simulink model "adc5g_r2_counter"  (Simulink 7.6)
settings: Solver=ode45  StartTime=0.0  StopTime=10.0  RelTol=1e-3
libraries: xbsIndex_r4 x22, simulink x16, dspsigops x16, xps_library x2, casper_library_misc x1
settings Model: Creator=rprimian  LastModifiedBy=rprimian
settings DebuggingCC: SolverPrmCheckMsg=none  StrictBusMsg=Warning

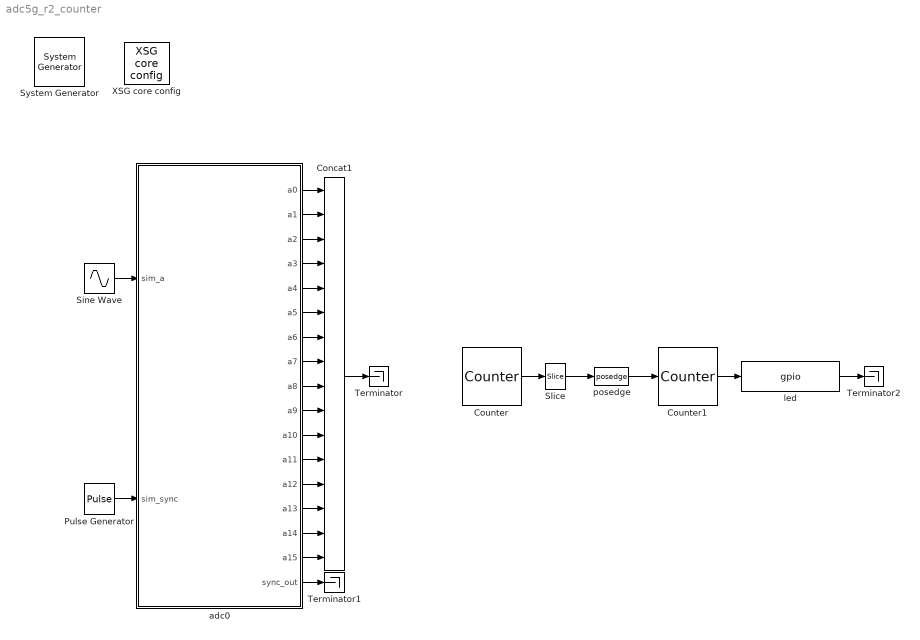
== system adc5g_r2_counter ==
  " System Generator" : xbsIndex_r4/ System Generator  Tag=genX  SystemSampleTime=-1  xilinxfamily=virtex6  part=xc6vsx475t  speed=-1  package=ff1759  synthesis_tool=XST  clock_wrapper=Clock Enables  directory=./adc5g_r2_counter/sysgen  proj_type=Project Navigator  testbench=off  simulink_period=1  sysclk_period=8  dcm_input_clock_period=100  incr_netlist=off  trim_vbits=Everywhere in SubSystem  dbl_ovrd=According to Block Masks  core_generation=According to Block Masks  run_coregen=off  deprecated_control=off  eval_field=0  block_type=sysgen
      settings: block_version=11.4
  Concat1 : xbsIndex_r4/Concat  num_inputs=16  dbl_ovrd=off  block_type=concat
  Counter : xbsIndex_r4/Counter  cnt_type=Free Running  cnt_to=Inf  operation=Up  start_count=0  cnt_by_val=1  arith_type=Unsigned  n_bits=32  bin_pt=0  load_pin=off  rst=off  en=off  explicit_period=on  period=1  dbl_ovrd=off  use_behavioral_HDL=off  implementation=Fabric  block_type=counter
  Counter1 : xbsIndex_r4/Counter  cnt_type=Free Running  cnt_to=Inf  operation=Up  start_count=0  cnt_by_val=1  arith_type=Unsigned  n_bits=8  bin_pt=0  load_pin=off  rst=off  en=on  explicit_period=on  period=1  dbl_ovrd=off  use_behavioral_HDL=off  implementation=Fabric  block_type=counter
  Pulse Generator : DiscretePulseGenerator  Period=1000
  Sine Wave : Sin  SineType=Sample based  SampleTime=1/8
  Slice : xbsIndex_r4/Slice  nbits=1  boolean_output=on  mode=Upper Bit Location + Width  bit1=-2  base1=MSB of Input  bit0=0  base0=LSB of Input  dbl_ovrd=off  block_type=slice
  Terminator : Terminator
  Terminator1 : Terminator
  Terminator2 : Terminator
  XSG core config : xps_library/XSG core config  Tag=xps:xsg  SystemSampleTime=-1  hw_sys=ROACH2:sx475t  ibob_linux=off  clk_src=adc0_clk  iBOB_clk_src=sys_clk  BEE2_ctrl_clk_src=sys_clk  BEE2_usr_clk_src=sys_clk  ROACH_clk_src=adc0_clk  ROACH2_clk_src=adc0_clk  CORR_clk_src=sys_clk  gpio_clk_io_group=iBOB:sma  gpio_clk_bit_index=0  clk_rate=125  sample_period=1  synthesis_tool=XST  mpc_type=powerpc440_ext
  adc0 : Subsystem  Tag=xps:adc5g  AncestorBlock=xps_library/ADCs/asiaa_adc5g  mask(adc5g){input_mode=One-channel -- A, adc_brd=ZDOK 0, demux=1:1, adc_bit_width=8, adc_clk_rate=1000, using_ctrl=on, test_ramp=off}
      mask prompts: input_mode "Input mode:"; adc_brd "ADC Board"; demux "Internal demux"; adc_bit_width "ADC Resolution (bits):"; adc_clk_rate "ADC Clock Rate (MHz):"; using_ctrl "use control"; test_ramp "start in test ramp mode"
      mask help:
      | Interface for the ASIAA 5 GSps ADC. Supports interleaving all four
      | cores using either input A or C, or interleaving two-cores each for
      | A and C. The hardware itself comes in two versions:
      |
      | DMUX 1:2 -- 4-bit samples, 4 parallel streams
      | DMUX 1:1 -- 8-bit samples, 2 parallel streams
      |
      | In either configuration this block will output 8 parallel streams
      | but the underlying interface, and the bitwidth of the samples,
      | will be different.
      mask init:
      | adc5g_init(gcb,...
      |     'input_mode', input_mode,...
      |     'demux', demux,...
      |     'adc_clk_rate', adc_clk_rate,...
      |     'adc_bit_width', adc_bit_width,...
      |     'adc_brd', adc_brd,...
      |     'using_ctrl', using_ctrl,...
      |     'test_ramp', test_ramp);
      mask StyleString: popup(One-channel -- A|One-channel -- C|Two-channel -- A&C),popup(ZDOK 0|ZDOK 1),popup(1:1|1:2),edit,edit,checkbox,checkbox
      mask CallbackString:
      | ||demux = get_param(gcb,'demux');
      | if(strcmp(demux,'1:1')),
      |     set_param(gcb, 'adc_bit_width', '8')
      | elseif(strcmp(demux, '1:2')),
      |     set_param(gcb, 'adc_bit_width', '4');
      | else
      | end||||
  led : xps_library/gpio  Tag=xps:gpio  SystemSampleTime=-1  io_group=ROACH2:led  io_dir=out  arith_type=Unsigned  bitwidth=8  bin_pt=0  bit_index=[0 1 2 3 4 5 6 7]  sample_period=1  use_single_ended=off  use_ddr=off  reg_iob=on  reg_clk_phase=0  termination=None
      link override convert: arith_type=Boolean  n_bits=8  bin_pt=0
  posedge : casper_library_misc/posedge  Tag=Rising Edge Detector  SystemSampleTime=-1
  wires:
  Pulse Generator/1 -> adc0/2(sim_sync)
  Concat1/1 -> Terminator/1
  Sine Wave/1 -> adc0/1(sim_a)
  adc0/1(a0) -> Concat1/1
  adc0/2(a1) -> Concat1/2
  adc0/3(a2) -> Concat1/3
  adc0/4(a3) -> Concat1/4
  adc0/5(a4) -> Concat1/5
  adc0/6(a5) -> Concat1/6
  adc0/7(a6) -> Concat1/7
  adc0/8(a7) -> Concat1/8
  adc0/9(a8) -> Concat1/9
  adc0/10(a9) -> Concat1/10
  adc0/11(a10) -> Concat1/11
  adc0/12(a11) -> Concat1/12
  adc0/13(a12) -> Concat1/13
  adc0/14(a13) -> Concat1/14
  adc0/15(a14) -> Concat1/15
  adc0/16(a15) -> Concat1/16
  adc0/17(sync_out) -> Terminator1/1
  Counter/1 -> Slice/1
  Slice/1 -> posedge/1
  led/1 -> Terminator2/1
  Counter1/1 -> led/1
  posedge/1 -> Counter1/1

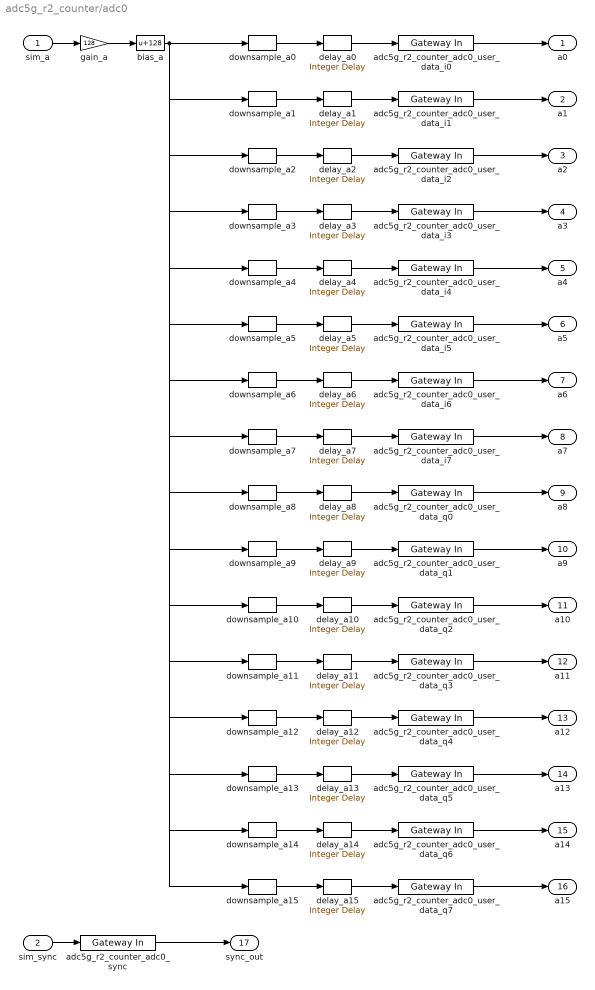
== system adc5g_r2_counter/adc0 ==
  sim_a : Inport
  sim_sync : Inport  Port=2
  adc5g_r2_counter_adc0_sync : xbsIndex_r4/Gateway In  arith_type=Boolean  n_bits=16  bin_pt=14  quantization="Round  (unbiased: +/- Inf)"  overflow=Saturate  period=1  dbl_ovrd=off  timing_constraint=None  locs_specified=off  LOCs={}  hdl_port=on  block_type=gatewayin
      settings: infoedit="Gateway in block.  Converts inputs of type Simulink integer, double and fixed point to  Xilinx fixed point type.<br><br>Hardware notes:  In hardware these blocks become top level input ports."
  adc5g_r2_counter_adc0_user_data_i{0..7} (8 alike) : xbsIndex_r4/Gateway In  arith_type=Unsigned  n_bits=8  bin_pt=0  quantization=Truncate  overflow=Wrap  period=1  dbl_ovrd=off  timing_constraint=None  locs_specified=off  LOCs={}  hdl_port=on  block_type=gatewayin
      settings: infoedit="Gateway in block.  Converts inputs of type Simulink integer, double and fixed point to  Xilinx fixed point type.<br><br>Hardware notes:  In hardware these blocks become top level input ports."
  adc5g_r2_counter_adc0_user_data_q{0..7} (8 alike) : xbsIndex_r4/Gateway In  arith_type=Unsigned  n_bits=8  bin_pt=0  quantization=Truncate  overflow=Wrap  period=1  dbl_ovrd=off  timing_constraint=None  locs_specified=off  LOCs={}  hdl_port=on  block_type=gatewayin
      settings: infoedit="Gateway in block.  Converts inputs of type Simulink integer, double and fixed point to  Xilinx fixed point type.<br><br>Hardware notes:  In hardware these blocks become top level input ports."
  bias_a : Bias  Bias=128  SaturateOnIntegerOverflow=on
  delay_a0 : simulink/Discrete/Integer Delay  NumDelays=2  InputProcessing=Inherited  vinit=0  samptime=-1
  delay_a{1..15} (15 alike) : simulink/Discrete/Integer Delay  NumDelays=1  InputProcessing=Inherited  vinit=0  samptime=-1
  downsample_a0 : dspsigops/Downsample  N=16  phase=0  InputProcessing=Inherited (this choice will be removed - see release notes)  RateOptions=Enforce single-rate processing  smode=Allow multirate  fmode=Maintain input frame size  ic=0
  downsample_a1 : dspsigops/Downsample  N=16  phase=1  InputProcessing=Inherited (this choice will be removed - see release notes)  RateOptions=Enforce single-rate processing  smode=Allow multirate  fmode=Maintain input frame size  ic=0
  downsample_a10 : dspsigops/Downsample  N=16  phase=10  InputProcessing=Inherited (this choice will be removed - see release notes)  RateOptions=Enforce single-rate processing  smode=Allow multirate  fmode=Maintain input frame size  ic=0
  downsample_a11 : dspsigops/Downsample  N=16  phase=11  InputProcessing=Inherited (this choice will be removed - see release notes)  RateOptions=Enforce single-rate processing  smode=Allow multirate  fmode=Maintain input frame size  ic=0
  downsample_a12 : dspsigops/Downsample  N=16  phase=12  InputProcessing=Inherited (this choice will be removed - see release notes)  RateOptions=Enforce single-rate processing  smode=Allow multirate  fmode=Maintain input frame size  ic=0
  downsample_a13 : dspsigops/Downsample  N=16  phase=13  InputProcessing=Inherited (this choice will be removed - see release notes)  RateOptions=Enforce single-rate processing  smode=Allow multirate  fmode=Maintain input frame size  ic=0
  downsample_a14 : dspsigops/Downsample  N=16  phase=14  InputProcessing=Inherited (this choice will be removed - see release notes)  RateOptions=Enforce single-rate processing  smode=Allow multirate  fmode=Maintain input frame size  ic=0
  downsample_a15 : dspsigops/Downsample  N=16  phase=15  InputProcessing=Inherited (this choice will be removed - see release notes)  RateOptions=Enforce single-rate processing  smode=Allow multirate  fmode=Maintain input frame size  ic=0
  downsample_a2 : dspsigops/Downsample  N=16  phase=2  InputProcessing=Inherited (this choice will be removed - see release notes)  RateOptions=Enforce single-rate processing  smode=Allow multirate  fmode=Maintain input frame size  ic=0
  downsample_a3 : dspsigops/Downsample  N=16  phase=3  InputProcessing=Inherited (this choice will be removed - see release notes)  RateOptions=Enforce single-rate processing  smode=Allow multirate  fmode=Maintain input frame size  ic=0
  downsample_a4 : dspsigops/Downsample  N=16  phase=4  InputProcessing=Inherited (this choice will be removed - see release notes)  RateOptions=Enforce single-rate processing  smode=Allow multirate  fmode=Maintain input frame size  ic=0
  downsample_a5 : dspsigops/Downsample  N=16  phase=5  InputProcessing=Inherited (this choice will be removed - see release notes)  RateOptions=Enforce single-rate processing  smode=Allow multirate  fmode=Maintain input frame size  ic=0
  downsample_a6 : dspsigops/Downsample  N=16  phase=6  InputProcessing=Inherited (this choice will be removed - see release notes)  RateOptions=Enforce single-rate processing  smode=Allow multirate  fmode=Maintain input frame size  ic=0
  downsample_a7 : dspsigops/Downsample  N=16  phase=7  InputProcessing=Inherited (this choice will be removed - see release notes)  RateOptions=Enforce single-rate processing  smode=Allow multirate  fmode=Maintain input frame size  ic=0
  downsample_a8 : dspsigops/Downsample  N=16  phase=8  InputProcessing=Inherited (this choice will be removed - see release notes)  RateOptions=Enforce single-rate processing  smode=Allow multirate  fmode=Maintain input frame size  ic=0
  downsample_a9 : dspsigops/Downsample  N=16  phase=9  InputProcessing=Inherited (this choice will be removed - see release notes)  RateOptions=Enforce single-rate processing  smode=Allow multirate  fmode=Maintain input frame size  ic=0
  gain_a : Gain  Gain=128  SaturateOnIntegerOverflow=on  OutDataTypeStr=Inherit: Same as input  ParamDataTypeStr=Inherit: Same as input
  a0 : Outport
  a1 : Outport  Port=2
  a2 : Outport  Port=3
  a3 : Outport  Port=4
  a4 : Outport  Port=5
  a5 : Outport  Port=6
  a6 : Outport  Port=7
  a7 : Outport  Port=8
  a8 : Outport  Port=9
  a9 : Outport  Port=10
  a10 : Outport  Port=11
  a11 : Outport  Port=12
  a12 : Outport  Port=13
  a13 : Outport  Port=14
  a14 : Outport  Port=15
  a15 : Outport  Port=16
  sync_out : Outport  Port=17
  wires:
  sim_a/1 -> gain_a/1
  gain_a/1 -> bias_a/1
  bias_a/1 -> downsample_a0/1, downsample_a1/1, downsample_a2/1, downsample_a3/1, downsample_a4/1, downsample_a5/1, downsample_a6/1, downsample_a7/1, downsample_a8/1, downsample_a9/1, downsample_a10/1, downsample_a11/1, downsample_a12/1, downsample_a13/1, downsample_a14/1, downsample_a15/1
  downsample_a0/1 -> delay_a0/1
  delay_a0/1 -> adc5g_r2_counter_adc0_user_data_i0/1
  adc5g_r2_counter_adc0_user_data_i0/1 -> a0/1
  downsample_a1/1 -> delay_a1/1
  delay_a1/1 -> adc5g_r2_counter_adc0_user_data_i1/1
  adc5g_r2_counter_adc0_user_data_i1/1 -> a1/1
  downsample_a2/1 -> delay_a2/1
  delay_a2/1 -> adc5g_r2_counter_adc0_user_data_i2/1
  adc5g_r2_counter_adc0_user_data_i2/1 -> a2/1
  downsample_a3/1 -> delay_a3/1
  delay_a3/1 -> adc5g_r2_counter_adc0_user_data_i3/1
  adc5g_r2_counter_adc0_user_data_i3/1 -> a3/1
  downsample_a4/1 -> delay_a4/1
  delay_a4/1 -> adc5g_r2_counter_adc0_user_data_i4/1
  adc5g_r2_counter_adc0_user_data_i4/1 -> a4/1
  downsample_a5/1 -> delay_a5/1
  delay_a5/1 -> adc5g_r2_counter_adc0_user_data_i5/1
  adc5g_r2_counter_adc0_user_data_i5/1 -> a5/1
  downsample_a6/1 -> delay_a6/1
  delay_a6/1 -> adc5g_r2_counter_adc0_user_data_i6/1
  adc5g_r2_counter_adc0_user_data_i6/1 -> a6/1
  downsample_a7/1 -> delay_a7/1
  delay_a7/1 -> adc5g_r2_counter_adc0_user_data_i7/1
  adc5g_r2_counter_adc0_user_data_i7/1 -> a7/1
  downsample_a8/1 -> delay_a8/1
  delay_a8/1 -> adc5g_r2_counter_adc0_user_data_q0/1
  adc5g_r2_counter_adc0_user_data_q0/1 -> a8/1
  downsample_a9/1 -> delay_a9/1
  delay_a9/1 -> adc5g_r2_counter_adc0_user_data_q1/1
  adc5g_r2_counter_adc0_user_data_q1/1 -> a9/1
  downsample_a10/1 -> delay_a10/1
  delay_a10/1 -> adc5g_r2_counter_adc0_user_data_q2/1
  adc5g_r2_counter_adc0_user_data_q2/1 -> a10/1
  downsample_a11/1 -> delay_a11/1
  delay_a11/1 -> adc5g_r2_counter_adc0_user_data_q3/1
  adc5g_r2_counter_adc0_user_data_q3/1 -> a11/1
  downsample_a12/1 -> delay_a12/1
  delay_a12/1 -> adc5g_r2_counter_adc0_user_data_q4/1
  adc5g_r2_counter_adc0_user_data_q4/1 -> a12/1
  downsample_a13/1 -> delay_a13/1
  delay_a13/1 -> adc5g_r2_counter_adc0_user_data_q5/1
  adc5g_r2_counter_adc0_user_data_q5/1 -> a13/1
  downsample_a14/1 -> delay_a14/1
  delay_a14/1 -> adc5g_r2_counter_adc0_user_data_q6/1
  adc5g_r2_counter_adc0_user_data_q6/1 -> a14/1
  downsample_a15/1 -> delay_a15/1
  delay_a15/1 -> adc5g_r2_counter_adc0_user_data_q7/1
  adc5g_r2_counter_adc0_user_data_q7/1 -> a15/1
  sim_sync/1 -> adc5g_r2_counter_adc0_sync/1
  adc5g_r2_counter_adc0_sync/1 -> sync_out/1
